simulink model "FmModulation"  (R2015a)
settings: Solver=ode45  StartTime=0.0  StopTime=10.0  RelTol=1e-3
settings Model: Creator=Chayti  LastModifiedBy=Chayti

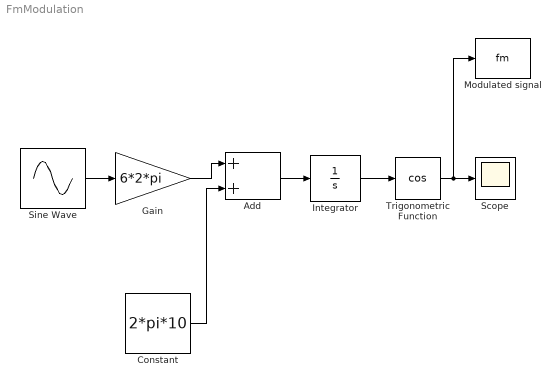
== system FmModulation ==
  Add : Sum
  Constant : Constant  Value=2*pi*10
  Gain : Gain  Gain=6*2*pi
  Integrator : Integrator
  Modulated signal : ToWorkspace  VariableName=fm  SaveFormat=Timeseries  SampleTime=-1
  Scope : Scope
  Sine Wave : Sin  Frequency=2*pi  Phase=pi/2  SampleTime=1/5000
  Trigonometric Function : Trigonometry  Operator=cos
  wires:
  Sine Wave/1 -> Gain/1
  Gain/1 -> Add/1
  Constant/1 -> Add/2
  Add/1 -> Integrator/1
  Integrator/1 -> Trigonometric Function/1
  Trigonometric Function/1 -> Modulated signal/1, Scope/1
